simulink model "HumanoidWalkerRobot"  (R2025b)
settings: Solver=daessc  StartTime=0.0  StopTime=params.simulation.Tf  RelTol=1e-3  AbsTol=1e-3
model workspace: external: MATLAB File sm_humanoid_walker_rl_parameters.m (data not in the file)
undefined symbols (not defined in the file): params, X, Y, Z
libraries: sm_lib x4, sm_humanoid_walker_lib x3, Humanoid_RL_Lib x2, nesl_utility x1, rllib x1
settings Model: Creator=The MathWorks, Inc.  LastModifiedBy=jolson
settings SolverCC: AlgebraicLoopSolver=TrustRegion
settings DebuggingCC: ParameterPrecisionLossMsg=none  ParameterTunabilityLossMsg=none  UnconnectedInputMsg=warning  UnconnectedOutputMsg=warning  UnconnectedLineMsg=warning
settings ModelReferenceCC: EnableRefExpFcnMdlSchedulingChecks=on
settings RTWCC: GPUComputeCapability=3.5  DLArmComputeVersion=19.05
settings ExplorerConfigSet: InternalSimMechanicsExplorerSettings="<ExplorerConfiguration><canonicalview>default</canonicalview><AnimationSetting><BasePlaybackSpeed>1.0</BasePlaybackSpeed><PlaybackSpeedFactor>1.0</PlaybackSpeedFactor></AnimationSetting><TilePanel><TileInfo><Tiles Columns=\"1\" Count=\"1\" Rows=\"1\"><Column Weight=\"1\"/><Row Weight=\"1\"/><Tile Height=\"1\" Width=\"1\" X=\"0\" Y=\"0\"/></Tiles></TileInfo><SceneInfo><SceneViewer><BGColor><R>0.800000011920928955</R><G>1</G><B>1</B></BGColor><Camera><DoPerspective>off</DoPerspective><Position><X>8.96755038464133847</X><Y>-33.9547954334831275</Y><Z>5.68566711732064345</Z></Position><Center><X>-1.58062354338744759</X><Y>-10.8119634269059119</Y><Z>1.15371617138283433</Z></Center><Up><X>-0.0712658071760212952</X><Y>0.160306311529002654</Y><Z>0.984491275335397265</Z></Up><ViewLimDist>1</ViewLimDist><YLim>4.18067302558725906</YLim><XLim>5.48162800275541695</XLim></Camera></SceneViewer></SceneInfo></TilePanel><MechEditorPanel><Cameras><Camera><Id>Camera1</Id><Value><Name>Camera1</Name><NativeCamera><PositionTrackingFeature>Humanoid_Walker.Humanoid_Robot_6_Joint.Camera_Frame.R</PositionTrackingFeature><CenterTrackingFeature>Humanoid_Walker.Humanoid_Robot_6_Joint.Aim_Frame.R</CenterTrackingFeature><UpVectorTrackingFeature>Humanoid_Walker.Humanoid_Robot_6_Joint.World.W</UpVectorTrackingFeature><CenterTrackingOrigin>on</CenterTrackingOrigin><UpVectorTrackingDirection>+Z</UpVectorTrackingDirection></NativeCamera></Value></Camera></Cameras><GfxPanelCameraMap/><VideoCreator><PlaybackSpeedRatio>1.0</PlaybackSpeedRatio><FrameRate>30</FrameRate><VideoFormat>Motion JPEG AVI</VideoFormat><FrameSize>auto</FrameSize></VideoCreator></MechEditorPanel></ExplorerConfiguration>"

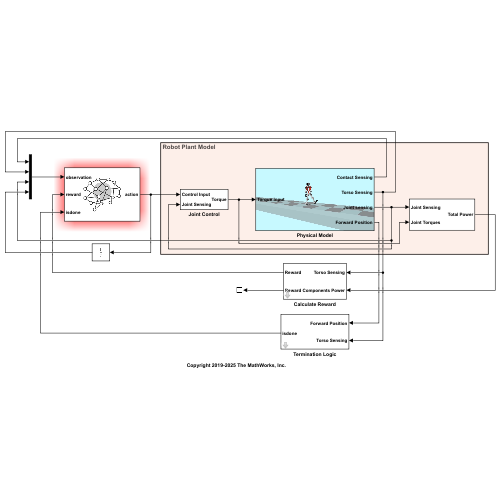
[thumbnail: Simulink's stored preview of the top-level diagram]
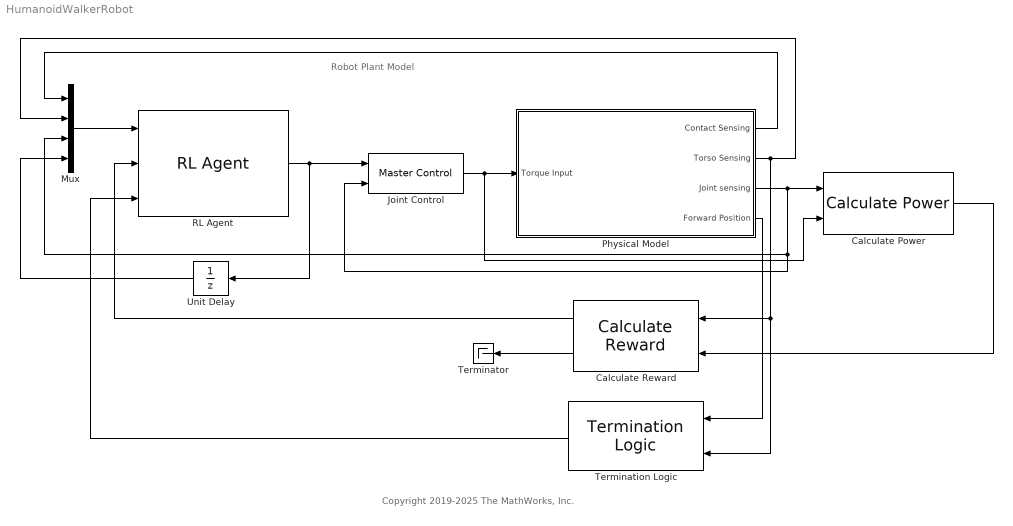
== system HumanoidWalkerRobot ==
  note: Robot Plant Model
  note: Copyright 2019-2025 The MathWorks, Inc.
  Calculate Power : sm_humanoid_walker_lib/Calculate Power  SystemSampleTime=-1  VariantActivationTime=update diagram  EmptyChoice=off  PassThrough=off  PassThroughVariantControl=(default)  EmptyChoiceVariantControl=(default)  AllowFlexibleInterface=on  Latency=0  AutoFrameSizeCalculation=off
  Calculate Reward : Humanoid_RL_Lib/Calculate Reward  forwardReward=params.reward.forwardRewardWeight  timestepReward=params.reward.timestepRewardWeight  powerPenalty=params.reward.powerPenaltyWeight  verticalPenalty=params.reward.verticalPenaltyWeight  lateralPenalty=params.reward.lateralPenaltyWeight
  Joint Control : sm_humanoid_walker_lib/Master Control  SystemSampleTime=-1  VariantActivationTime=update diagram  EmptyChoice=off  PassThrough=off  PassThroughVariantControl=(default)  EmptyChoiceVariantControl=(default)  AllowFlexibleInterface=on  Latency=0  AutoFrameSizeCalculation=off
  Mux : Mux
  Physical Model : Subsystem
      mask Display: image('imagebackground.PNG'); % Use "Edit Image" on toolstrip to change.
  RL Agent : rllib/RL Agent  Agent=agentObj  ExternalActionAsInput=off  ProvideLastAction=off  ProvideCumRwd=off  TreatAsDirectFeedthrough=on  UseStrictObservationDataTypes=off
  Termination Logic : Humanoid_RL_Lib/Termination Logic  verticalStop=params.stoppingCriteria.heightChange  lateralStop=params.stoppingCriteria.lateral  angularStop=params.stoppingCriteria.angle  timeoutTime=params.stoppingCriteria.timeoutTime  timeoutDistance=params.stoppingCriteria.timeoutDistance
  Terminator : Terminator
  Unit Delay : UnitDelay  SampleTime=-1  HasFrameUpgradeWarning=on
  wires:
  Joint Control/1 -> Calculate Power/2, Physical Model/1(Torque Input)
  Physical Model/3(Joint sensing) -> Mux/3, Joint Control/2, Calculate Power/1
  Physical Model/2(Torso Sensing) -> Termination Logic/2, Calculate Reward/1, Mux/2
  Calculate Power/1 -> Calculate Reward/2
  Physical Model/4(Forward Position) -> Termination Logic/1
  RL Agent/1 -> Joint Control/1, Unit Delay/1
  Mux/1 -> RL Agent/1
  Physical Model/1(Contact Sensing) -> Mux/1
  Unit Delay/1 -> Mux/4
  Calculate Reward/1 -> RL Agent/2
  Calculate Reward/2 -> Terminator/1
  Termination Logic/1 -> RL Agent/3

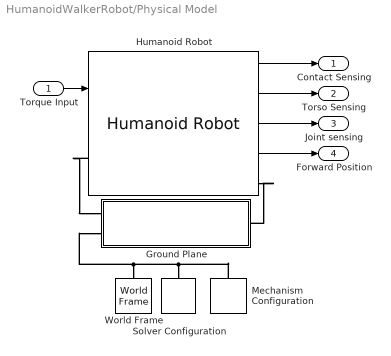
== system HumanoidWalkerRobot/Physical Model ==
  Torque Input : Inport
  Ground Plane : Subsystem
  Humanoid Robot : sm_humanoid_walker_lib/Humanoid Robot  contactRadius=params.contact.contactRadius  contactStiffness=params.contact.stiffness  contactDamping=params.contact.damping  contactTWidth=params.contact.transitionWidth  contactStaticFriction=params.contact.staticFriction  contactDynamicFriction=params.contact.dynamicFriction  contactCriticalVelocity=params.contact.criticalVelocity  footDensity=params.materialProperties.lowerBodyDensity  lowerLegDensity=params.materialProperties.lowerBodyDensity  upperLegDensity=params.materialProperties.lowerBodyDensity  hipDensity=params.materialProperties.lowerBodyDensity  trunkDensity=params.materialProperties.upperBodyDensity  shoulderDensity=params.materialProperties.upperBodyDensity  upperArmDensity=params.materialProperties.upperBodyDensity  lowerArmDensity=params.materialProperties.upperBodyDensity  handDensity=params.materialProperties.upperBodyDensity  headDensity=params.materialProperties.upperBodyDensity  hipUpperLimit=params.jointLimits.hipFrontalUpperLimit  hipLowerLimit=params.jointLimits.hipFrontalLowerLimit  kneeUpperLimit=params.jointLimits.kneeUpperLimit  kneeLowerLimit=params.jointLimits.kneeLowerLimit  ankleUpperLimit=params.jointLimits.ankleUpperLimit  ankleLowerLimit=params.jointLimits.ankleLowerLimit  shoulderFrontalUpperLimit=params.jointLimits.shoulderFrontalUpperLimit  shoulderFrontalLowerLimit=params.jointLimits.shoulderFrontalLowerLimit  shoulderSagittalUpperLimit=params.jointLimits.shoulderSagittalUpperLimit  shoulderSagittalLowerLimit=params.jointLimits.shoulderSagittalLowerLimit
  Mechanism Configuration : sm_lib/Utilities/Mechanism Configuration  UniformGravity=Constant  GravityVector=[0 0 -9.80665]  GravityVectorUnits=m/s^2  LinearizationDelta=0.001  JointModeTransitionNonlinearIterations=2
  Solver Configuration : nesl_utility/Solver Configuration  PhysicalDomain=network_engine_domain  SubClassName=solver  LeftPortType=input  RightPortType=generic  Tones=[]  Harmonics=[]  SimulateNoise=off  Profile=off  UseLocalSampling=off  EnableSwitchedLinearOptims=on  FrequencyDomain=off  UseCCode=off  RelTol=0.001  AbsTol=1e-06  MinStep=1e-09  ToWorkspace=off  RevertToSquareIcSolve=off  NumHomotopyIterations=100  PhasorMode=off  PhasorModeNumHarmonics=1  ConsistencySolver=NEWTON_FTOL  IndexReductionMethod=DerivativeReplacement  DoDC=off  ResidualTolerance=1e-09  ConsistencyTolSource=GLOBAL  ConsistencyAbsTol=0.001  ConsistencyRelTol=0.001  ConsistencyTolFactor=0.001  UseLocalSolver=off  LocalSolverChoice=NE_BACKWARD_EULER_ADVANCER  ResolveIndetEquations=on  FunctionEvalNumThread=1  LocalSolverSampleTime=0.001  DoFixedCost=off  MaxNonlinIter=3  MaxModeIter=2  ComputeImpulses=off  ImpulseIterations=2  LinearAlgebra=auto  LinearAlgebraNumThread=0  EquationFormulation=NE_TIME_EF  DelaysMemoryBudget=1024  AutomaticFiltering=on  FilteringTimeConstant=0.001  PartitionStorageMethod=AS_NEEDED  PartitionMemoryBudget=1024  PartitionMethod=ROBUST  MultibodyUseLocalSolver=off  MultibodyLocalSolverChoice=ODE1  MultibodyLocalSolverSampleTime=0.001
  World Frame : sm_lib/Frames and Transforms/World Frame
  Contact Sensing : Outport
  Torso Sensing : Outport  Port=2
  Joint sensing : Outport  Port=3
  Forward Position : Outport  Port=4
  wires:
  Humanoid Robot/2 -> Torso Sensing/1
  Humanoid Robot/1 -> Contact Sensing/1
  Torque Input/1 -> Humanoid Robot/1
  Humanoid Robot/3 -> Joint sensing/1
  Humanoid Robot/4 -> Forward Position/1
  connections:
  Humanoid Robot/RConn1 -- Ground Plane/RConn1
  Mechanism Configuration/RConn1 -- World Frame/RConn1 -- Ground Plane/LConn2 -- Solver Configuration/RConn1
  Humanoid Robot/LConn1 -- Ground Plane/LConn1

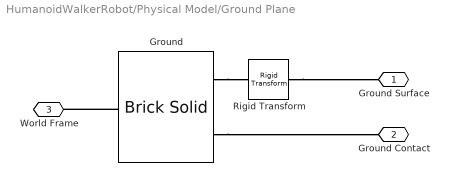
== system HumanoidWalkerRobot/Physical Model/Ground Plane ==
  Ground : sm_lib/Body Elements/Brick Solid  BrickDimensions=[params.display.planeWidth params.display.planeLength params.display.planeHeight]  BrickDimensionsUnits=m  ExportEntireGeometry=on  InertiaType=CalculateFromGeometry  BasedOnType=Density  Density=1000  DensityUnits=kg/m^3  Mass=1  MassUnits=kg  CenterOfMass=[0 0 0]  CenterOfMassUnits=m  MomentsOfInertia=[1 1 1]  MomentsOfInertiaUnits=kg*m^2  ProductsOfInertia=[0 0 0]  ProductsOfInertiaUnits=kg*m^2  GraphicType=FromGeometry  MarkerShape=Sphere  MarkerSize=10  GraphicVisPropType=SimpleVisualProperties  GraphicDiffuseColor=params.display.floorColour  GraphicOpacity=0.3  GraphicSpecularColor=[0.5 0.5 0.5 1.0]  GraphicAmbientColor=[0.15 0.15 0.15 1.0]  GraphicEmissiveColor=[0.0 0.0 0.0 1.0]  GraphicShininess=75  DoExposeReferenceFrame=on  SerializedFrames=<Frames><Frame><Id>Frame1</Id><Value><Name>GS</Name><Origin><Source>GeometricFeature</Source><FeatureName>+z surface</FeatureName></Origin><PrimaryAxis><DefinedDirection>+Z</DefinedDirection><Source>ReferenceFrame</Source><SourceDirection>+Z</SourceDirection><FeatureName></FeatureName></PrimaryAxis><SecondaryAxis><DefinedDirection>+X</DefinedDirection><Source>ReferenceFrame</Source><SourceDirection>+X</SourceDirection><FeatureName></FeatureName></SecondaryAxis></Value></Frame></Frames>
  Rigid Transform : sm_lib/Frames and Transforms/Rigid Transform  RotationMethod=None  FollAlignAxisA=+X  BaseAlignAxisA=+Y  FollAlignAxisB=+Y  BaseAlignAxisB=+Z  RotationStandardAxis=+Z  RotationAngle=0.0  RotationAngleUnits=deg  RotationArbitraryAxis=[0 0 1]  RotationSequenceAxes=FollowerAxes  RotationSequence=XYX  RotationSequenceAngles=[0 0 0]  RotationSequenceAnglesUnits=deg  RotationMatrix=[1 0 0; 0 1 0; 0 0 1]  Quaternion=[1 0 0 0]  TranslationMethod=StandardAxis  TranslationCartesianOffset=[0 0 0]  TranslationCartesianOffsetUnits=m  TranslationStandardAxis=+Y  TranslationStandardOffset=0.5-(params.display.planeLength/2)  TranslationStandardOffsetUnits=m  TranslationROffset=0  TranslationROffsetUnits=m  TranslationThetaOffset=0  TranslationThetaOffsetUnits=deg  TranslationZOffset=0  TranslationZOffsetUnits=m
  Ground Surface : PMIOPort  Side=Left
  Ground Contact : PMIOPort  Port=2  Side=Right
  World Frame : PMIOPort  Port=3  Side=Left
  connections:
  Ground/LConn1 -- Rigid Transform/LConn1
  Ground/LConn2 -- Ground Contact/RConn1
  Ground/RConn1 -- World Frame/RConn1
  Rigid Transform/RConn1 -- Ground Surface/RConn1
